simulink model "MSFartoystyring1_2018"  (R2018b)
settings: Solver=ode45  StartTime=tstart  StopTime=tstop  RelTol=1e-3  EnableMultiTasking=on
values from neighbouring files (symbols this model uses):
  c = 0    [nomoto1.m]    (also in run.m)
  delta_c = 10*pi/180    (= 0.174532925199)    [nomoto1.m]    (also in run.m)
  K = n/d(2)    [nomoto1.m]
  Kd = 127.2314    [run.m]
  Ki = 0.022    [run.m]
  Kp = 2.5446    [run.m]
  n_c = 7.3    [nomoto1.m]    (also in run.m)
  p0 = zeros(2,1)    [nomoto1.m]    (also in run.m)
  psi0 = 0    [nomoto1.m]    (also in run.m)
  r0 = 0    [nomoto1.m]    (also in run.m)
  T = 1/d(2)    [nomoto1.m]
  tsamp = 1    [nomoto1.m]    (also in run.m)
  v0 = [6.63 0]'    [nomoto1.m]    (also in run.m)
undefined symbols (not defined in the file or in its folder): msfartoystyring
settings Model: ExtModeAutoUpdateStatusClock=off  Creator=christh  LastModifiedBy=ola
settings DataIOCC: LimitDataPoints=on  SaveFormat=Array  SignalLoggingSaveFormat=ModelDataLogs
settings OptimizationCC: ExpressionDepthLimit=2147483647  InitFltsAndDblsToZero=on  LifeSpan=inf
settings DebuggingCC: UnderspecifiedInitializationDetection=Classic  MergeDetectMultiDrivingBlocksExec=none  SolverPrmCheckMsg=warning  FcnCallInpInsideContextMsg=warning  StateNameClashWarn=warning  SFUnexpectedBacktrackingDiag=warning  SFNoUnconditionalDefaultTransitionDiag=warning
settings HardwareCC: ProdBitPerPointer=32  ProdBitPerSizeT=32  ProdBitPerPtrDiffT=32  ProdLargestAtomicFloat=None  ProdIntDivRoundTo=Undefined  ProdEndianess=Unspecified  ProdWordSize=32  ProdHWDeviceType=32-bit Generic
settings ModelReferenceCC: PropagateSignalLabelsOutOfModel=off
settings SFSimCC: SimUseLocalCustomCode=off
settings RTWCC: RTWUseLocalCustomCode=off
settings CodeAppCC: StateflowObjectComments=on
settings GRTTargetCC: TargetLangStandard=C89/C90 (ANSI)  GeneratePreprocessorConditionals=Disable all  CombineOutputUpdateFcns=off  GRTInterface=on
settings ConfigComp: CovMetricSettings=dw  CovHtmlReporting=on  CovSaveCumulativeToWorkspaceVar=on  CovSaveSingleToWorkspaceVar=on  CovExternalEMLEnable=off

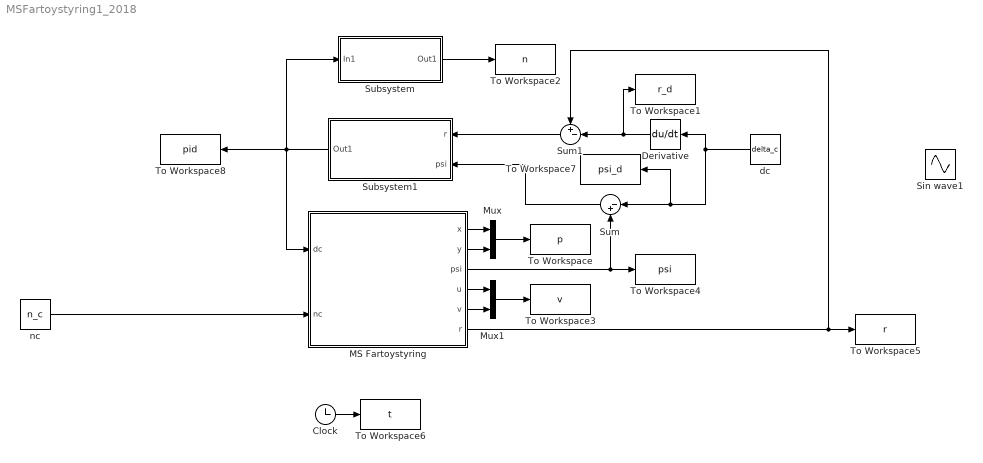
== system MSFartoystyring1_2018 ==
  Clock : Clock
  Derivative : Derivative
  MS Fartoystyring : Subsystem  mask(MS Fartoystyring for Assignment 3 G&C){x0=p0(1), y0=p0(2), u0=v0(1), v0=v0(2), psi0=psi0, r0=r0, c=c}
      mask prompts: x0 "x(t0) (m)"; y0 "y(t0) (m)"; u0 "u(t0) (m/s)"; v0 "v(t0) (m/s)"; psi0 "psi(t0) (rad)"; r0 "r(t0) (rad/s)"; c "current (0 or 1)"
      mask help:
      | Block corresponding to Figure 1 in the assignment text. Gives the response of the ship.
      |
      | The design speed of MS Fartoystyring is u=8.23 m/s.
      |
      | Input:
      | dc: commanded rudder (rad), dmax=25*pi/180
      | nc: commanded shaft speed (rad/s), nmax=85*2*pi/60
      |
      | Output:
      | x: north pos (m)
      | y: east pos (m)
      | u: surge (m/s)
      | v: sway (m/s)
      | psi: heading (rad)
      | r: yaw (rad/s)
      mask Help: Comments, bugs and help requests can be directed to the TA. Email on course website.
  Mux : Mux  Inputs=2
  Mux1 : Mux  Inputs=2
  Sin wave1 : Sin  Amplitude=0.4  Frequency=0.004  SampleTime=0
  Subsystem : Subsystem
  Subsystem1 : Subsystem
  Sum : Sum  Inputs=|-+
  Sum1 : Sum  Inputs=+-|
  To Workspace : ToWorkspace  VariableName=p  SampleTime=tsamp
  To Workspace1 : ToWorkspace  VariableName=r_d  SampleTime=tsamp
  To Workspace2 : ToWorkspace  VariableName=n  SampleTime=tsamp
  To Workspace3 : ToWorkspace  VariableName=v  SampleTime=tsamp
  To Workspace4 : ToWorkspace  VariableName=psi  SampleTime=tsamp
  To Workspace5 : ToWorkspace  VariableName=r  SampleTime=tsamp
  To Workspace6 : ToWorkspace  VariableName=t  SampleTime=tsamp
  To Workspace7 : ToWorkspace  VariableName=psi_d  SampleTime=tsamp
  To Workspace8 : ToWorkspace  VariableName=pid  SampleTime=tsamp
  dc : Constant  Value=delta_c
  nc : Constant  Value=n_c
  wires:
  Clock/1 -> To Workspace6/1
  MS Fartoystyring/1(x) -> Mux/1
  MS Fartoystyring/2(y) -> Mux/2
  MS Fartoystyring/4(u) -> Mux1/1
  MS Fartoystyring/5(v) -> Mux1/2
  Mux/1 -> To Workspace/1
  Mux1/1 -> To Workspace3/1
  nc/1 -> MS Fartoystyring/2(nc)
  MS Fartoystyring/3(psi) -> Sum/2, To Workspace4/1
  Subsystem/1(Out1) -> To Workspace2/1
  Subsystem1/1(Out1) -> To Workspace8/1, MS Fartoystyring/1(dc), Subsystem/1(In1)
  Sum/1 -> Subsystem1/2(psi)
  Sum1/1 -> Subsystem1/1(r)
  MS Fartoystyring/6(r) -> To Workspace5/1, Sum1/1
  dc/1 -> Derivative/1, To Workspace7/1, Sum/1
  Derivative/1 -> Sum1/2, To Workspace1/1

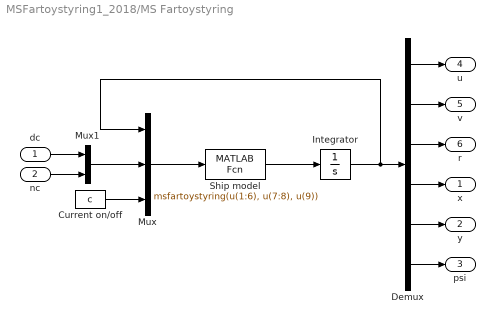
== system MSFartoystyring1_2018/MS Fartoystyring ==
  dc : Inport
  nc : Inport  Port=2
  Current on/off : Constant  Value=c
  Demux : Demux  Outputs=6
  Integrator : Integrator  InitialCondition=[u0 v0 r0 x0 y0 psi0]'
  Mux : Mux  Inputs=3
  Mux1 : Mux  Inputs=2
  Ship model : MATLABFcn  MATLABFcn=msfartoystyring(u(1:6), u(7:8), u(9))  OutputDimensions=6
  x : Outport
  y : Outport  Port=2
  psi : Outport  Port=3
  u : Outport  Port=4
  v : Outport  Port=5
  r : Outport  Port=6
  wires:
  Integrator/1 -> Mux/1, Demux/1
  Mux1/1 -> Mux/2
  dc/1 -> Mux1/1
  nc/1 -> Mux1/2
  Demux/1 -> u/1
  Demux/2 -> v/1
  Demux/3 -> r/1
  Demux/4 -> x/1
  Demux/5 -> y/1
  Demux/6 -> psi/1
  Current on/off/1 -> Mux/3
  Ship model/1 -> Integrator/1
  Mux/1 -> Ship model/1

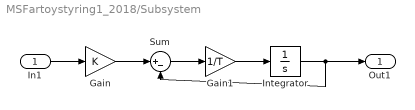
== system MSFartoystyring1_2018/Subsystem ==
  In1 : Inport
  Gain : Gain  Gain=K
  Gain1 : Gain  Gain=1/T
  Integrator : Integrator
  Sum : Sum  Inputs=|+-
  Out1 : Outport
  wires:
  In1/1 -> Gain/1
  Gain/1 -> Sum/1
  Gain1/1 -> Integrator/1
  Sum/1 -> Gain1/1
  Integrator/1 -> Sum/2, Out1/1

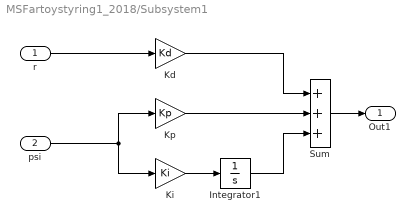
== system MSFartoystyring1_2018/Subsystem1 ==
  r : Inport
  psi : Inport  Port=2
  Integrator1 : Integrator
  Kd : Gain  Gain=Kd
  Ki : Gain  Gain=Ki
  Kp : Gain  Gain=Kp
  Sum : Sum  Inputs=+++
  Out1 : Outport
  wires:
  r/1 -> Kd/1
  Sum/1 -> Out1/1
  psi/1 -> Ki/1, Kp/1
  Ki/1 -> Integrator1/1
  Integrator1/1 -> Sum/3
  Kp/1 -> Sum/2
  Kd/1 -> Sum/1
